simulink model "Vehicle_definitivo_validazione_2"  (R2025b)
settings: Solver=ode4  StartTime=0.0  StopTime=30  FixedStep=0.001  RelTol=1e-3
undefined symbols (not defined in the file): car, new_lotus_bump, new_lotus_roll, new_lotus_steer, posRef, rad, s, Tau_1, Tau_2, Tau_3, Tau_4, yawRef
libraries: aerolibconvert2 x28, simulink_extras x16, simulink x12, slpidlib x2, mpclib x1
(part 5 of 13)

== system Vehicle_definitivo_validazione_2/Torque Vectoring/Vehicle/Powertrain/Electric Motor ==
  T_target : Inport
  omega wheels : Inport  Port=2
  Angular Velocity Conversion : aerolibconvert2/Angular Velocity Conversion  IU=rpm  OU=rad/s
  Angular Velocity Conversion1 : aerolibconvert2/Angular Velocity Conversion  IU=rad/s  OU=rpm
  Angular Velocity Conversion2 : aerolibconvert2/Angular Velocity Conversion  IU=rpm  OU=rad/s
  Demux : Demux
  Gain1 : Gain  Gain=car.Tau_EM
  Gain2 : Gain  Gain=car.Tau_EM
  Gain3 : Gain  Gain=car.Tau_EM
  Integrator : Integrator  InitialCondition=1  LimitOutput=on  UpperSaturationLimit=1  LowerSaturationLimit=0
  Limiter1 : Saturate  UpperLimit=16000  LowerLimit=0
  MATLAB Function : MATLAB Function  TreatAsAtomicUnit=on
  MATLAB Function1 : MATLAB Function  TreatAsAtomicUnit=on
  Torque+ : Lookup_n-D  NumberOfTableDimensions=1  BreakpointsForDimension1=[0;5415.9399999999996;5455.8699999999999;5494.6300000000001;5524.8000000000002;5801.2200000000003;6194.8599999999997;6620.2799999999997;6996.5;7478.6599999999999;8072.5500000000002;8891.9799999999996;8998.9200000000001;9966.8600000000006;10994.200000000001;11872.6;13016.16;13972.65;15994.85]  Table=[6.914188;6.910217;6.868869;6.845731;6.823144;6.614154;6.313463;6.000783;5.723209;5.399066;4.994964;4.498184;4.450257;3.941032;3.52511;3.198601;2.816719;2.558901;2.040423]  InternalRulePriority=Speed  RndMeth=Simplest
  Torque+1 : Lookup_n-D  NumberOfTableDimensions=1  BreakpointsForDimension1=[0;5415.9399999999996;5455.8699999999999;5494.6300000000001;5524.8000000000002;5801.2200000000003;6194.8599999999997;6620.2799999999997;6996.5;7478.6599999999999;8072.5500000000002;8891.9799999999996;8998.9200000000001;9966.8600000000006;10994.200000000001;11872.6;13016.16;13972.65;15994.85]  Table=[6.914188;6.910217;6.868869;6.845731;6.823144;6.614154;6.313463;6.000783;5.723209;5.399066;4.994964;4.498184;4.450257;3.941032;3.52511;3.198601;2.816719;2.558901;2.040423]  InternalRulePriority=Speed  RndMeth=Simplest
  Torque- : Lookup_n-D  NumberOfTableDimensions=1  BreakpointsForDimension1=[0;5415.9399999999996;5455.8699999999999;5494.6300000000001;5524.8000000000002;5801.2200000000003;6194.8599999999997;6620.2799999999997;6996.5;7478.6599999999999;8072.5500000000002;8891.9799999999996;8998.9200000000001;9966.8600000000006;10994.200000000001;11872.6;13016.16;13972.65;15994.85]  Table=-[6.914188;6.910217;6.868869;6.845731;6.823144;6.614154;6.313463;6.000783;5.723209;5.399066;4.994964;4.498184;4.450257;3.941032;3.52511;3.198601;2.816719;2.558901;2.040423]  InternalRulePriority=Speed  RndMeth=Simplest
  Torque-1 : Lookup_n-D  NumberOfTableDimensions=1  BreakpointsForDimension1=[0;5415.9399999999996;5455.8699999999999;5494.6300000000001;5524.8000000000002;5801.2200000000003;6194.8599999999997;6620.2799999999997;6996.5;7478.6599999999999;8072.5500000000002;8891.9799999999996;8998.9200000000001;9966.8600000000006;10994.200000000001;11872.6;13016.16;13972.65;15994.85]  Table=-[6.914188;6.910217;6.868869;6.845731;6.823144;6.614154;6.313463;6.000783;5.723209;5.399066;4.994964;4.498184;4.450257;3.941032;3.52511;3.198601;2.816719;2.558901;2.040423]  InternalRulePriority=Speed  RndMeth=Simplest
  T_FR : Outport
  T_FL : Outport  Port=2
  wires:
  omega wheels/1 -> Angular Velocity Conversion1/1
  Angular Velocity Conversion1/1 -> Gain3/1
  Gain3/1 -> Limiter1/1
  Limiter1/1 -> Demux/1
  Demux/1 -> Torque+/1, Torque-/1, Angular Velocity Conversion/1
  Demux/2 -> Torque-1/1, Angular Velocity Conversion2/1, Torque+1/1
  MATLAB Function/1(SoC_dot) -> Integrator/1
  Integrator/1 -> MATLAB Function/5(SoC)
  Angular Velocity Conversion/1 -> MATLAB Function/3(w_FR)
  Angular Velocity Conversion2/1 -> MATLAB Function/4(w_FL)
  Torque+/1 -> MATLAB Function1/2(T_max_pos_FR)  "T_FR+"
  Torque+1/1 -> MATLAB Function1/4(T_max_pos_FL)  "T_FL+"
  Torque-/1 -> MATLAB Function1/3(T_max_neg_FR)  "T_FR-"
  Torque-1/1 -> MATLAB Function1/5(T_max_neg_FL)  "T_FL-"
  T_target/1 -> MATLAB Function1/1(T_target)
  MATLAB Function1/2(T_actual_FL) -> Gain2/1, MATLAB Function/2(T_FL)
  MATLAB Function1/1(T_actual_FR) -> Gain1/1, MATLAB Function/1(T_FR)
  Gain1/1 -> T_FR/1
  Gain2/1 -> T_FL/1

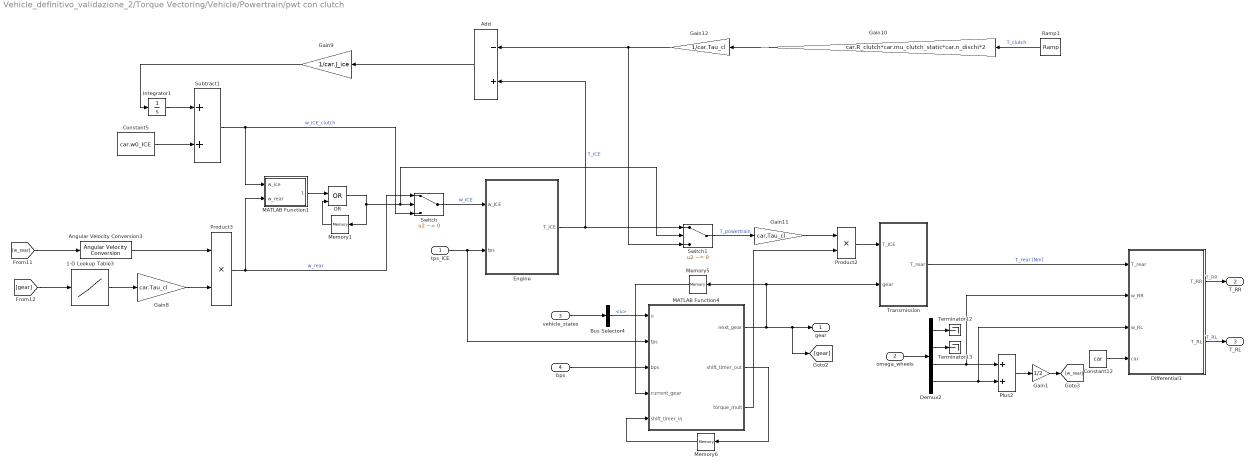
== system Vehicle_definitivo_validazione_2/Torque Vectoring/Vehicle/Powertrain/pwt con clutch ==
  tps_ICE : Inport
  omega_wheels : Inport  Port=2
  vehicle_states : Inport  Port=3
  bps : Inport  Port=4
  1-D Lookup Table3 : Lookup_n-D  NumberOfTableDimensions=1  BreakpointsForDimension1=[1;2;3;4]  Table=[Tau_1; Tau_2; Tau_3; Tau_4]  InternalRulePriority=Speed  RndMeth=Simplest
  Add : Sum  Inputs=-+
  Angular Velocity Conversion3 : aerolibconvert2/Angular Velocity Conversion  IU=rad/s  OU=rpm
  Bus Selector4 : BusSelector  OutputSignals=velocities.u
  Constant12 : Constant  Value=car  OutDataTypeStr=Bus: slBus1
  Constant5 : Constant  Value=car.w0_ICE
  Demux2 : Demux
  Differential1 : MATLAB Function  TreatAsAtomicUnit=on
  Engine : Subsystem
  Gain1 : Gain  Gain=1/2
  Gain10 : Gain  Gain=car.R_clutch*car.mu_clutch_static*car.n_dischi*2
  Gain11 : Gain  Gain=car.Tau_cl
  Gain12 : Gain  Gain=1/car.Tau_cl
  Gain8 : Gain  Gain=car.Tau_cl
  Gain9 : Gain  Gain=1/car.J_ice
  Integrator1 : Integrator
  MATLAB Function1 : MATLAB Function  TreatAsAtomicUnit=on
  MATLAB Function4 : MATLAB Function  TreatAsAtomicUnit=on
  Memory1 : Memory
  Memory5 : Memory  InitialCondition=2
  Memory6 : Memory
  OR : Logic  Operator=OR  IconShape=distinctive  AllPortsSameDT=off  OutDataTypeStr=boolean
  Plus2 : Sum
  Product2 : Product
  Product3 : Product
  Ramp1 : simulink/Sources/Ramp  slope=5000  start=0  InitialOutput=671
  Subtract1 : Sum
  Switch : Switch  Criteria=u2 ~= 0  Threshold=50  SaturateOnIntegerOverflow=off  InputSameDT=off
  Switch1 : Switch  Criteria=u2 ~= 0  Threshold=50  SaturateOnIntegerOverflow=off  InputSameDT=off
  Terminator12 : Terminator
  Terminator13 : Terminator
  Transmission : Subsystem
  gear : Outport
  T_RR : Outport  Port=2
  T_RL : Outport  Port=3
  wires:
  Ramp1/1 -> Gain10/1  "T_clutch"
  MATLAB Function1/1(condizione) -> OR/1
  [gear] -> 1-D Lookup Table3/1
  Gain10/1 -> Gain12/1
  Angular Velocity Conversion3/1 -> Product3/1
  [w_rear] -> Angular Velocity Conversion3/1
  Gain12/1 -> Switch1/3, Add/1
  Integrator1/1 -> Subtract1/1
  Switch/1 -> Engine/1(w_ICE)  "w_ICE"
  Subtract1/1 -> Switch/3, MATLAB Function1/1(w_ice)  "w_ICE_clutch"
  Switch1/1 -> Gain11/1  "T_powertrain"
  Constant5/1 -> Subtract1/2
  Memory1/1 -> OR/2
  tps_ICE/1 -> Engine/2(tps), MATLAB Function4/2(tps)
  Add/1 -> Gain9/1
  Memory5/1 -> MATLAB Function4/4(current_gear)
  bps/1 -> MATLAB Function4/3(bps)
  OR/1 -> Memory1/1, Switch/2, Switch1/2
  vehicle_states/1 -> Bus Selector4/1
  Demux2/1 -> Terminator12/1
  Gain8/1 -> Product3/2
  Gain1/1 -> [w_rear]
  1-D Lookup Table3/1 -> Gain8/1
  Plus2/1 -> Gain1/1
  omega_wheels/1 -> Demux2/1
  MATLAB Function4/2(shift_timer_out) -> Memory6/1
  Transmission/1(T_rear) -> Differential1/1(T_rear)  "T_rear [Nm]"
  Memory6/1 -> MATLAB Function4/5(shift_timer_in)
  Demux2/2 -> Terminator13/1
  Demux2/4 -> Differential1/3(w_RL), Plus2/2
  Bus Selector4/1 -> MATLAB Function4/1(u)  "<u>"
  Demux2/3 -> Differential1/2(w_RR), Plus2/1
  MATLAB Function4/1(next_gear) -> Memory5/1, Transmission/2(gear), gear/1, [gear]
  Product3/1 -> MATLAB Function1/2(w_rear), Switch/1  "w_rear"
  Gain11/1 -> Product2/1
  MATLAB Function4/3(torque_mult) -> Product2/2
  Engine/1(T_ICE) -> Add/2, Switch1/1  "T_ICE"
  Gain9/1 -> Integrator1/1
  Product2/1 -> Transmission/1(T_ICE)
  Differential1/1(T_RR) -> T_RR/1  "T_RR"
  Constant12/1 -> Differential1/4(car)
  Differential1/2(T_RL) -> T_RL/1  "T_RL"

== system Vehicle_definitivo_validazione_2/Torque Vectoring/Vehicle/Powertrain/pwt senza clutch ==
  tps_ICE : Inport
  vehicle_states : Inport  Port=2
  bps : Inport  Port=3
  omega_wheels : Inport  Port=4
  1-D Lookup Table1 : Lookup_n-D  NumberOfTableDimensions=1  BreakpointsForDimension1=[1;2;3;4]  Table=[Tau_1; Tau_2; Tau_3; Tau_4]  InternalRulePriority=Speed  RndMeth=Simplest
  Angular Velocity Conversion1 : aerolibconvert2/Angular Velocity Conversion  IU=rad/s  OU=rpm
  Bus Selector3 : BusSelector  OutputSignals=Veh_States.velocities.u
  Constant12 : Constant  Value=car  OutDataTypeStr=Bus: slBus1
  Demux : Demux
  Differential : MATLAB Function  TreatAsAtomicUnit=on
  Engine : Subsystem
  Gain1 : Gain  Gain=1/2
  Gain2 : Gain  Gain=car.Tau_cl
  Gain5 : Gain  Gain=car.Tau_cl
  Gearbox : MATLAB Function  TreatAsAtomicUnit=on
  Memory : Memory  InitialCondition=2
  Memory3 : Memory
  Plus : Sum
  Product : Product
  Product1 : Product
  Terminator : Terminator
  Terminator1 : Terminator
  Transmission : Subsystem
  T_RR : Outport
  T_RL : Outport  Port=2
  gear : Outport  Port=3
  wires:
  Memory/1 -> Gearbox/4(current_gear)
  Gain5/1 -> Product1/2
  vehicle_states/1 -> Bus Selector3/1
  Angular Velocity Conversion1/1 -> Product1/1
  Gearbox/3(shift_timer_out) -> Memory3/1
  Memory3/1 -> Gearbox/5(shift_timer_in)
  bps/1 -> Gearbox/3(bps)  "bps"
  1-D Lookup Table1/1 -> Gain5/1
  Bus Selector3/1 -> Gearbox/1(u)  "<u>"
  Gearbox/1(next_gear) -> Memory/1, Transmission/2(gear), gear/1, [gear]  "gear"
  [gear] -> 1-D Lookup Table1/1
  Transmission/1(T_rear) -> Differential/1(T_rear)  "T_rear [Nm]"
  tps_ICE/1 -> Gearbox/2(tps), Engine/2(tps)  "tps"
  Product/1 -> Transmission/1(T_ICE)
  Engine/1(T_ICE) -> Gain2/1  "T_ICE"
  Product1/1 -> Engine/1(w_ICE)  "w_ICE"
  Gearbox/2(torque_mult) -> Product/2
  Gain2/1 -> Product/1
  Plus/1 -> Gain1/1
  Demux/3 -> Plus/1, [w_RR]
  Gain1/1 -> Angular Velocity Conversion1/1
  Demux/4 -> [w_RL], Plus/2
  omega_wheels/1 -> Demux/1
  Demux/1 -> Terminator/1  "w_front"
  Demux/2 -> Terminator1/1
  Differential/1(T_RR) -> T_RR/1  "T_RR"
  Differential/2(T_RL) -> T_RL/1  "T_RL"
  [w_RR] -> Differential/2(w_RR)
  [w_RL] -> Differential/3(w_RL)
  Constant12/1 -> Differential/4(car)

== system Vehicle_definitivo_validazione_2/Torque Vectoring/Vehicle/Powertrain con differenziale1/Electric Motor ==
  tps_EM : Inport
  omega wheels : Inport  Port=2
  2-D Lookup Table : Lookup_n-D  BreakpointsForDimension1=[0;5415.9399999999996;5455.8699999999999;5494.6300000000001;5524.8000000000002;5801.2200000000003;6194.8599999999997;6620.2799999999997;6996.5;7478.6599999999999;8072.5500000000002;8891.9799999999996;8998.9200000000001;9966.8600000000006;10994.200000000001;11872.6;13016.16;13972.65;15994.85]  BreakpointsForDimension2=[0;0.25;0.29999999999999999;0.34999999999999998;0.40000000000000002;0.45000000000000001;0.5;0.59999999999999998;0.69999999999999996;0.80000000000000004;1]  Table=[0 1.72854705 2.07425646 2.41996587 2.7656752899999999 3.1113846999999999 3.4570941099999999 4.1485129299999999 4.8399317000000002 5.5313505699999999 6.9141880000000002;0 1.72755429 2.0730651500000001 2.4185760100000002 2.7640868599999999 3.10959772 3.4551085800000001 4.1461303000000003 4.8371519999999997 5.5281737299999998 6.9102170000000003;0 1.7172173399999999 2.0606608099999999 2.4041042799999999 2.7475477499999998 3.0909912099999999 3.4344346799999999 4.1213216199999998 4.8082086000000004 5.4950954899999997 6.8688690000000001;0 1.7114327 2.0537192399999999 2.3960057799999999 2.7382923199999998 3.0805788600000001 3.4228654000000001 4.1074384799999999 4.7920116000000004 5.4765846399999996 6.8457309999999998;0 1.7057860899999999 2.0469433100000001 2.3881005200000001 2.72925774 3.0704149599999999 3.4115721799999998 4.0938866100000002 4.7762010000000004 5.45851548 6.8231440000000001;0 1.65353861 1.9842463299999999 2.3149540499999999 2.6456617699999998 2.9763694900000002 3.3070772100000001 3.96849265 4.6299080999999997 5.2913235399999996 6.6141540000000001;0 1.57836584 1.89403901 2.2097121799999999 2.5253853500000001 2.8410585199999998 3.15673168 3.7880780199999999 4.4194243999999996 5.0507707000000002 6.3134629999999996;0 1.5001957400000001 1.80023489 2.10027404 2.4003131899999999 2.7003523399999998 3.0003914800000002 3.6004697800000001 4.2005480999999998 4.8006263699999998 6.0007830000000002;0 1.43080228 1.71696274 2.0031231900000002 2.2892836499999998 2.5754440999999999 2.86160456 3.4339254700000001 4.0062464000000002 4.5785672899999996 5.7232089999999998;0 1.34976662 1.6197199499999999 1.8896732700000001 2.1596266000000002 2.4295799200000001 2.69953325 3.2394398899999999 3.7793464999999999 4.3192531900000004 5.3990660000000004;0 1.24874098 1.49848917 1.74823737 1.99798556 2.24773376 2.4974819500000001 2.9969783400000001 3.4964746999999998 3.9959711200000001 4.9949640000000004;0 1.1245459799999999 1.3494551800000001 1.57436438 1.79927357 2.0241827699999999 2.2490919699999998 2.6989103600000002 3.1487288000000002 3.5985471499999999 4.4981840000000002;0 1.11256427 1.3350771299999999 1.5575899799999999 1.7801028299999999 2.0026156899999998 2.22512854 2.67015425 3.1151800000000001 3.5602056700000002 4.4502569999999997;0 0.98525799000000003 1.18230959 1.3793611800000001 1.5764127800000001 1.7734643800000001 1.9705159800000001 2.3646191700000001 2.7587223999999999 3.1528255600000001 3.9410319999999999;0 0.88127745999999996 1.0575329600000001 1.23378845 1.41004394 1.5862994399999999 1.7625549300000001 2.1150659100000002 2.4675769000000001 2.8200878899999999 3.5251100000000002;0 0.79965012999999996 0.95958014999999997 1.11951018 1.2794402 1.43937023 1.59930025 1.9191602999999999 2.2390203999999998 2.5588804000000001 3.198601;0 0.70417978000000003 0.84501572999999996 0.98585168999999995 1.1266876400000001 1.2675236000000001 1.4083595600000001 1.6900314700000001 1.9717034 2.2533752900000001 2.816719;0 0.63972525999999996 0.76767032000000002 0.89561537000000002 1.0235604199999999 1.15150547 1.2794505300000001 1.5353406300000001 1.7912307000000001 2.0471208399999998 2.5589010000000001;0 0.51010575999999996 0.61212690999999997 0.71414805999999997 0.81616922000000003 0.91819037000000003 1.0202115199999999 1.2242538199999999 1.4282961000000001 1.6323384299999999 2.0404230000000001]  InternalRulePriority=Speed  RndMeth=Simplest
      settings: InputPortMap=u0,u1
  2-D Lookup Table1 : Lookup_n-D  BreakpointsForDimension1=[0;5415.9399999999996;5455.8699999999999;5494.6300000000001;5524.8000000000002;5801.2200000000003;6194.8599999999997;6620.2799999999997;6996.5;7478.6599999999999;8072.5500000000002;8891.9799999999996;8998.9200000000001;9966.8600000000006;10994.200000000001;11872.6;13016.16;13972.65;15994.85]  BreakpointsForDimension2=[0;0.25;0.29999999999999999;0.34999999999999998;0.40000000000000002;0.45000000000000001;0.5;0.59999999999999998;0.69999999999999996;0.80000000000000004;1]  Table=[0 1.72854705 2.07425646 2.41996587 2.7656752899999999 3.1113846999999999 3.4570941099999999 4.1485129299999999 4.8399317000000002 5.5313505699999999 6.9141880000000002;0 1.72755429 2.0730651500000001 2.4185760100000002 2.7640868599999999 3.10959772 3.4551085800000001 4.1461303000000003 4.8371519999999997 5.5281737299999998 6.9102170000000003;0 1.7172173399999999 2.0606608099999999 2.4041042799999999 2.7475477499999998 3.0909912099999999 3.4344346799999999 4.1213216199999998 4.8082086000000004 5.4950954899999997 6.8688690000000001;0 1.7114327 2.0537192399999999 2.3960057799999999 2.7382923199999998 3.0805788600000001 3.4228654000000001 4.1074384799999999 4.7920116000000004 5.4765846399999996 6.8457309999999998;0 1.7057860899999999 2.0469433100000001 2.3881005200000001 2.72925774 3.0704149599999999 3.4115721799999998 4.0938866100000002 4.7762010000000004 5.45851548 6.8231440000000001;0 1.65353861 1.9842463299999999 2.3149540499999999 2.6456617699999998 2.9763694900000002 3.3070772100000001 3.96849265 4.6299080999999997 5.2913235399999996 6.6141540000000001;0 1.57836584 1.89403901 2.2097121799999999 2.5253853500000001 2.8410585199999998 3.15673168 3.7880780199999999 4.4194243999999996 5.0507707000000002 6.3134629999999996;0 1.5001957400000001 1.80023489 2.10027404 2.4003131899999999 2.7003523399999998 3.0003914800000002 3.6004697800000001 4.2005480999999998 4.8006263699999998 6.0007830000000002;0 1.43080228 1.71696274 2.0031231900000002 2.2892836499999998 2.5754440999999999 2.86160456 3.4339254700000001 4.0062464000000002 4.5785672899999996 5.7232089999999998;0 1.34976662 1.6197199499999999 1.8896732700000001 2.1596266000000002 2.4295799200000001 2.69953325 3.2394398899999999 3.7793464999999999 4.3192531900000004 5.3990660000000004;0 1.24874098 1.49848917 1.74823737 1.99798556 2.24773376 2.4974819500000001 2.9969783400000001 3.4964746999999998 3.9959711200000001 4.9949640000000004;0 1.1245459799999999 1.3494551800000001 1.57436438 1.79927357 2.0241827699999999 2.2490919699999998 2.6989103600000002 3.1487288000000002 3.5985471499999999 4.4981840000000002;0 1.11256427 1.3350771299999999 1.5575899799999999 1.7801028299999999 2.0026156899999998 2.22512854 2.67015425 3.1151800000000001 3.5602056700000002 4.4502569999999997;0 0.98525799000000003 1.18230959 1.3793611800000001 1.5764127800000001 1.7734643800000001 1.9705159800000001 2.3646191700000001 2.7587223999999999 3.1528255600000001 3.9410319999999999;0 0.88127745999999996 1.0575329600000001 1.23378845 1.41004394 1.5862994399999999 1.7625549300000001 2.1150659100000002 2.4675769000000001 2.8200878899999999 3.5251100000000002;0 0.79965012999999996 0.95958014999999997 1.11951018 1.2794402 1.43937023 1.59930025 1.9191602999999999 2.2390203999999998 2.5588804000000001 3.198601;0 0.70417978000000003 0.84501572999999996 0.98585168999999995 1.1266876400000001 1.2675236000000001 1.4083595600000001 1.6900314700000001 1.9717034 2.2533752900000001 2.816719;0 0.63972525999999996 0.76767032000000002 0.89561537000000002 1.0235604199999999 1.15150547 1.2794505300000001 1.5353406300000001 1.7912307000000001 2.0471208399999998 2.5589010000000001;0 0.51010575999999996 0.61212690999999997 0.71414805999999997 0.81616922000000003 0.91819037000000003 1.0202115199999999 1.2242538199999999 1.4282961000000001 1.6323384299999999 2.0404230000000001]  InternalRulePriority=Speed  RndMeth=Simplest
      settings: InputPortMap=u0,u1
  Angular Velocity Conversion1 : aerolibconvert2/Angular Velocity Conversion  IU=rad/s  OU=rpm
  Demux : Demux
  Gain : Gain  Gain=car.Tau_EM
  Gain1 : Gain  Gain=car.Tau_EM
  Gain3 : Gain  Gain=car.Tau_EM
  Limiter1 : Saturate  UpperLimit=16000  LowerLimit=0
  T_FR : Outport
  T_FL : Outport  Port=2
  wires:
  Demux/2 -> 2-D Lookup Table1/1
  Demux/1 -> 2-D Lookup Table/1
  Limiter1/1 -> Demux/1
  tps_EM/1 -> 2-D Lookup Table/2, 2-D Lookup Table1/2
  Gain1/1 -> T_FL/1
  Gain/1 -> T_FR/1
  Gain3/1 -> Limiter1/1
  Angular Velocity Conversion1/1 -> Gain3/1
  omega wheels/1 -> Angular Velocity Conversion1/1
  2-D Lookup Table1/1 -> Gain1/1
  2-D Lookup Table/1 -> Gain/1

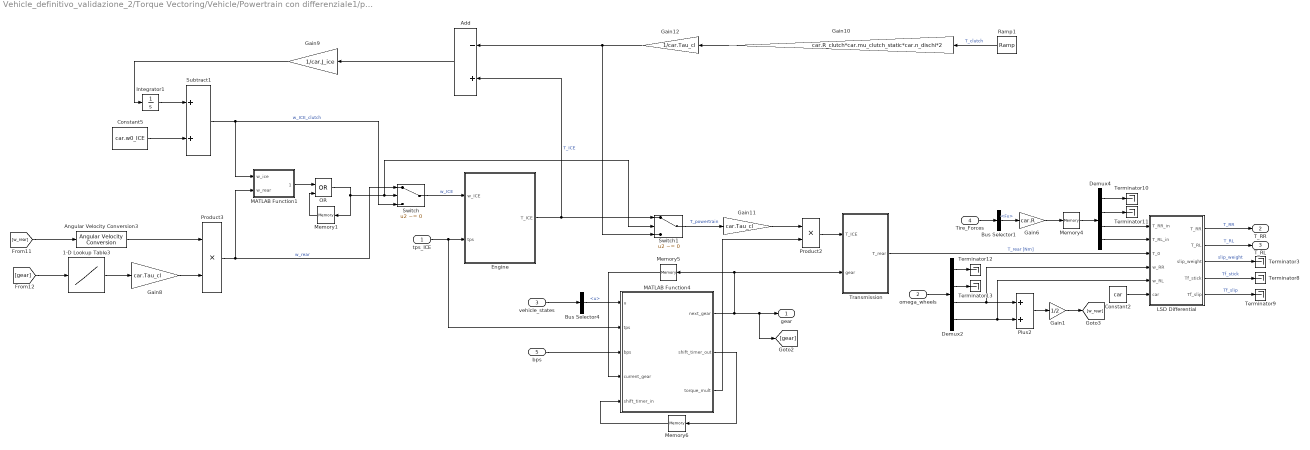
== system Vehicle_definitivo_validazione_2/Torque Vectoring/Vehicle/Powertrain con differenziale1/pwt con clutch ==
  tps_ICE : Inport
  omega_wheels : Inport  Port=2
  vehicle_states : Inport  Port=3
  Tire_Forces : Inport  Port=4
  bps : Inport  Port=5
  1-D Lookup Table3 : Lookup_n-D  NumberOfTableDimensions=1  BreakpointsForDimension1=[1;2;3;4]  Table=[Tau_1; Tau_2; Tau_3; Tau_4]  InternalRulePriority=Speed  RndMeth=Simplest
  Add : Sum  Inputs=-+
  Angular Velocity Conversion3 : aerolibconvert2/Angular Velocity Conversion  IU=rad/s  OU=rpm
  Bus Selector1 : BusSelector  OutputSignals=Fx
  Bus Selector4 : BusSelector  OutputSignals=velocities.u
  Constant2 : Constant  Value=car  OutDataTypeStr=Bus: slBus1
  Constant5 : Constant  Value=car.w0_ICE
  Demux2 : Demux
  Demux4 : Demux
  Engine : Subsystem
  Gain1 : Gain  Gain=1/2
  Gain10 : Gain  Gain=car.R_clutch*car.mu_clutch_static*car.n_dischi*2
  Gain11 : Gain  Gain=car.Tau_cl
  Gain12 : Gain  Gain=1/car.Tau_cl
  Gain6 : Gain  Gain=car.R
  Gain8 : Gain  Gain=car.Tau_cl
  Gain9 : Gain  Gain=1/car.J_ice
  Integrator1 : Integrator
  LSD Differential : MATLAB Function  TreatAsAtomicUnit=on
  MATLAB Function1 : MATLAB Function  TreatAsAtomicUnit=on
  MATLAB Function4 : MATLAB Function  TreatAsAtomicUnit=on
  Memory1 : Memory
  Memory4 : Memory
  Memory5 : Memory  InitialCondition=2
  Memory6 : Memory
  OR : Logic  Operator=OR  IconShape=distinctive  AllPortsSameDT=off  OutDataTypeStr=boolean
  Plus2 : Sum
  Product2 : Product
  Product3 : Product
  Ramp1 : simulink/Sources/Ramp  slope=5000  start=0  InitialOutput=671
  Subtract1 : Sum
  Switch : Switch  Criteria=u2 ~= 0  Threshold=50  SaturateOnIntegerOverflow=off  InputSameDT=off
  Switch1 : Switch  Criteria=u2 ~= 0  Threshold=50  SaturateOnIntegerOverflow=off  InputSameDT=off
  Terminator{3,8..13} (7 alike) : Terminator
  Transmission : Subsystem
  gear : Outport
  T_RR : Outport  Port=2
  T_RL : Outport  Port=3
  wires:
  Product2/1 -> Transmission/1(T_ICE)
  Demux4/1 -> Terminator10/1
  Gain9/1 -> Integrator1/1
  Engine/1(T_ICE) -> Switch1/1, Add/2  "T_ICE"
  MATLAB Function4/3(torque_mult) -> Product2/2
  Gain11/1 -> Product2/1
  LSD Differential/1(T_RR) -> T_RR/1  "T_RR"
  Product3/1 -> Switch/1, MATLAB Function1/2(w_rear)  "w_rear"
  Tire_Forces/1 -> Bus Selector1/1
  LSD Differential/4(Tf_stick) -> Terminator8/1  "Tf_stick"
  MATLAB Function4/1(next_gear) -> [gear], gear/1, Transmission/2(gear), Memory5/1
  Demux2/3 -> LSD Differential/4(w_RR), Plus2/1
  Bus Selector4/1 -> MATLAB Function4/1(u)  "<u>"
  Gain6/1 -> Memory4/1
  LSD Differential/5(Tf_slip) -> Terminator9/1  "Tf_slip"
  Demux4/4 -> LSD Differential/2(T_RL_in)
  LSD Differential/3(slip_weight) -> Terminator3/1  "slip_weight"
  Demux2/4 -> LSD Differential/5(w_RL), Plus2/2
  LSD Differential/2(T_RL) -> T_RL/1  "T_RL"
  Demux2/2 -> Terminator13/1
  Memory4/1 -> Demux4/1
  Constant2/1 -> LSD Differential/6(car)
  Memory6/1 -> MATLAB Function4/5(shift_timer_in)
  Demux4/3 -> LSD Differential/1(T_RR_in)
  Transmission/1(T_rear) -> LSD Differential/3(T_0)  "T_rear [Nm]"
  Bus Selector1/1 -> Gain6/1  "<Fx>"
  Demux4/2 -> Terminator11/1
  MATLAB Function4/2(shift_timer_out) -> Memory6/1
  omega_wheels/1 -> Demux2/1
  Plus2/1 -> Gain1/1
  1-D Lookup Table3/1 -> Gain8/1
  Gain1/1 -> [w_rear]
  Gain8/1 -> Product3/2
  Demux2/1 -> Terminator12/1
  vehicle_states/1 -> Bus Selector4/1
  OR/1 -> Switch1/2, Switch/2, Memory1/1
  bps/1 -> MATLAB Function4/3(bps)
  Memory5/1 -> MATLAB Function4/4(current_gear)
  Add/1 -> Gain9/1
  tps_ICE/1 -> MATLAB Function4/2(tps), Engine/2(tps)
  Memory1/1 -> OR/2
  Constant5/1 -> Subtract1/2
  Switch1/1 -> Gain11/1  "T_powertrain"
  Subtract1/1 -> MATLAB Function1/1(w_ice), Switch/3  "w_ICE_clutch"
  Switch/1 -> Engine/1(w_ICE)  "w_ICE"
  Integrator1/1 -> Subtract1/1
  Gain12/1 -> Add/1, Switch1/3
  [w_rear] -> Angular Velocity Conversion3/1
  Angular Velocity Conversion3/1 -> Product3/1
  Gain10/1 -> Gain12/1
  [gear] -> 1-D Lookup Table3/1
  MATLAB Function1/1(condizione) -> OR/1
  Ramp1/1 -> Gain10/1  "T_clutch"

== system Vehicle_definitivo_validazione_2/Torque Vectoring/Vehicle/Powertrain con differenziale1/pwt senza clutch ==
  tps_ICE : Inport
  omega_wheels : Inport  Port=2
  vehicle_states : Inport  Port=3
  Tire_Forces : Inport  Port=4
  bps : Inport  Port=5
  1-D Lookup Table1 : Lookup_n-D  NumberOfTableDimensions=1  BreakpointsForDimension1=[1;2;3;4]  Table=[Tau_1; Tau_2; Tau_3; Tau_4]  InternalRulePriority=Speed  RndMeth=Simplest
  Angular Velocity Conversion1 : aerolibconvert2/Angular Velocity Conversion  IU=rad/s  OU=rpm
  Bus Selector2 : BusSelector  OutputSignals=Fx
  Bus Selector3 : BusSelector  OutputSignals=velocities.u
  Constant1 : Constant  Value=car  OutDataTypeStr=Bus: slBus1
  Demux1 : Demux
  Demux3 : Demux
  Engine : Subsystem
  Gain2 : Gain  Gain=1/2
  Gain3 : Gain  Gain=car.R
  Gain4 : Gain  Gain=car.Tau_cl
  Gain5 : Gain  Gain=car.Tau_cl
  LSD Differential : MATLAB Function  TreatAsAtomicUnit=on
  MATLAB Function3 : MATLAB Function  TreatAsAtomicUnit=on
  Memory : Memory  InitialCondition=2
  Memory2 : Memory
  Memory3 : Memory
  Plus1 : Sum
  Product : Product
  Product1 : Product
  Terminator{,1..2,4..7} (7 alike) : Terminator
  Transmission : Subsystem
  T_RR : Outport
  T_RL : Outport  Port=2
  gear : Outport  Port=3
  wires:
  Gain4/1 -> Product/1
  MATLAB Function3/3(torque_mult) -> Product/2
  Product1/1 -> Engine/1(w_ICE)  "w_ICE"
  LSD Differential/4(Tf_stick) -> Terminator1/1  "Tf_stick"
  LSD Differential/5(Tf_slip) -> Terminator2/1  "Tf_slip"
  LSD Differential/3(slip_weight) -> Terminator/1  "slip_weight"
  Demux1/3 -> LSD Differential/4(w_RR), Plus1/1
  Engine/1(T_ICE) -> Gain4/1  "T_ICE"
  Demux1/4 -> LSD Differential/5(w_RL), Plus1/2
  Demux3/4 -> LSD Differential/2(T_RL_in)
  Demux1/2 -> Terminator7/1
  omega_wheels/1 -> Demux1/1
  Product/1 -> Transmission/1(T_ICE)
  [w_rear] -> Angular Velocity Conversion1/1
  Tire_Forces/1 -> Bus Selector2/1
  LSD Differential/2(T_RL) -> T_RL/1  "T_RL"
  Demux3/3 -> LSD Differential/1(T_RR_in)
  tps_ICE/1 -> Engine/2(tps), MATLAB Function3/2(tps)  "tps"
  Transmission/1(T_rear) -> LSD Differential/3(T_0)  "T_rear [Nm]"
  LSD Differential/1(T_RR) -> T_RR/1  "T_RR"
  [gear] -> 1-D Lookup Table1/1
  MATLAB Function3/1(next_gear) -> [gear], gear/1, Transmission/2(gear), Memory/1  "gear"
  Gain2/1 -> [w_rear]
  Bus Selector3/1 -> MATLAB Function3/1(u)  "<u>"
  Memory2/1 -> Demux3/1
  Constant1/1 -> LSD Differential/6(car)
  Demux3/1 -> Terminator4/1
  1-D Lookup Table1/1 -> Gain5/1
  Gain3/1 -> Memory2/1
  bps/1 -> MATLAB Function3/3(bps)  "bps"
  Memory3/1 -> MATLAB Function3/5(shift_timer_in)
  MATLAB Function3/2(shift_timer_out) -> Memory3/1
  Bus Selector2/1 -> Gain3/1  "<Fx>"
  Angular Velocity Conversion1/1 -> Product1/1
  Plus1/1 -> Gain2/1
  vehicle_states/1 -> Bus Selector3/1
  Gain5/1 -> Product1/2
  Demux3/2 -> Terminator5/1
  Memory/1 -> MATLAB Function3/4(current_gear)
  Demux1/1 -> Terminator6/1

== system Vehicle_definitivo_validazione_2/Con relaxation/Vehicle/Chassis/Damper/FL ==
  V_FL : Inport
  Add : Sum
  Add1 : Sum
  Add2 : Sum
  Front compression min : Lookup_n-D  NumberOfTableDimensions=1  BreakpointsForDimension1=|  Table=|  InternalRulePriority=Speed  RndMeth=Simplest
      BreakpointsForDimension1=|
      | [0;0.025;0.051;0.076;0.102;0.127;0.152;0.178;0.203;0.229;0.254;0.279;0.305
      | ]
      Table=|
      | [0; 240.204;
      | 231.307;
      | 226.859;
      | 226.859;
      | 231.307;
      | 231.307;
      | 235.756;
      | 240.204;
      | 240.204;
      | 244.652;
      | 249.100;
      | 253.549]
  Gain : Gain  Gain=-1
  Gain1 : Gain  Gain=-1
  Gain2 : Gain  Gain=car.click_comp_F/car.click_tot_comp_F
  Gain3 : Gain  Gain=car.click_reb_F/car.click_tot_reb_F
  Saturation : Saturate  UpperLimit=inf  LowerLimit=0
  Saturation1 : Saturate  UpperLimit=0  LowerLimit=-inf
  Subtract : Sum  Inputs=+-
  Subtract1 : Sum  Inputs=+-
  front compression max : Lookup_n-D  NumberOfTableDimensions=1  BreakpointsForDimension1=|  Table=|  InternalRulePriority=Speed  RndMeth=Simplest
      BreakpointsForDimension1=|
      | [0;0.025;0.051;0.076;0.102;0.127;0.152;0.178;0.203;0.229;0.254;0.279;0.305
      | ]
      Table=|
      | [0;782.887;
      | 898.540;
      | 956.367;
      | 978.608;
      | 1000.850;
      | 1018.642;
      | 1058.676;
      | 1085.366;
      | 1107.607;
      | 1147.641
      | ;1178.778;1214.364
      | ]
  front rebound max : Lookup_n-D  NumberOfTableDimensions=1  BreakpointsForDimension1=|  Table=|  InternalRulePriority=Speed  RndMeth=Simplest
      BreakpointsForDimension1=|
      | [0;0.025;0.051;0.076;0.102;0.127;0.152;0.178;0.203;0.229;0.254;0.279;0.305
      | ]
      Table=|
      | [0; 266.893;
      | 333.617;
      | 360.306;
      | 373.650;
      | 391.443;
      | 409.236;
      | 422.581;
      | 444.822;
      | 467.063;
      | 480.408;
      | 493.752;
      | 511.545]
  front rebound min : Lookup_n-D  NumberOfTableDimensions=1  BreakpointsForDimension1=|  Table=|  InternalRulePriority=Speed  RndMeth=Simplest
      BreakpointsForDimension1=|
      | [0;0.025;0.051;0.076;0.102;0.127;0.152;0.178;0.203;0.229;0.254;0.279;0.305
      | ]
      Table=|
      | [0; 40.034;
      | 26.689;
      | 17.793;
      | 8.896;
      | 4.448;
      | 4.448;
      | 4.448;
      | 8.896;
      | 35.586;
      | 31.138;
      | 53.379;
      | 26.689]
  F_FL : Outport
  wires:
  Front compression min/1 -> Subtract/2, Add1/2
  front rebound min/1 -> Add2/2, Subtract1/2
  Subtract1/1 -> Gain3/1
  Gain3/1 -> Add2/1
  Subtract/1 -> Gain2/1
  Gain2/1 -> Add1/1
  front compression max/1 -> Subtract/1
  front rebound max/1 -> Subtract1/1
  Saturation/1 -> front compression max/1, Front compression min/1
  Gain1/1 -> front rebound min/1, front rebound max/1
  Add2/1 -> Gain/1
  V_FL/1 -> Saturation/1, Saturation1/1
  Saturation1/1 -> Gain1/1
  Gain/1 -> Add/2
  Add1/1 -> Add/1
  Add/1 -> F_FL/1

== system Vehicle_definitivo_validazione_2/Con relaxation/Vehicle/Chassis/Damper/FR ==
  V_FR : Inport
  Add : Sum
  Add1 : Sum
  Add2 : Sum
  Front compression min : Lookup_n-D  NumberOfTableDimensions=1  BreakpointsForDimension1=|  Table=|  InternalRulePriority=Speed  RndMeth=Simplest
      BreakpointsForDimension1=|
      | [0;0.025;0.051;0.076;0.102;0.127;0.152;0.178;0.203;0.229;0.254;0.279;0.305
      | ]
      Table=|
      | [0; 240.204;
      | 231.307;
      | 226.859;
      | 226.859;
      | 231.307;
      | 231.307;
      | 235.756;
      | 240.204;
      | 240.204;
      | 244.652;
      | 249.100;
      | 253.549]
  Gain : Gain  Gain=-1
  Gain1 : Gain  Gain=-1
  Gain2 : Gain  Gain=car.click_comp_F/car.click_tot_comp_F
  Gain3 : Gain  Gain=car.click_reb_F/car.click_tot_reb_F
  Saturation : Saturate  UpperLimit=inf  LowerLimit=0
  Saturation1 : Saturate  UpperLimit=0  LowerLimit=-inf
  Subtract : Sum  Inputs=+-
  Subtract1 : Sum  Inputs=+-
  front compression max : Lookup_n-D  NumberOfTableDimensions=1  BreakpointsForDimension1=|  Table=|  InternalRulePriority=Speed  RndMeth=Simplest
      BreakpointsForDimension1=|
      | [0;0.025;0.051;0.076;0.102;0.127;0.152;0.178;0.203;0.229;0.254;0.279;0.305
      | ]
      Table=|
      | [0;782.887;
      | 898.540;
      | 956.367;
      | 978.608;
      | 1000.850;
      | 1018.642;
      | 1058.676;
      | 1085.366;
      | 1107.607;
      | 1147.641
      | ;1178.778;1214.364
      | ]
  front rebound max : Lookup_n-D  NumberOfTableDimensions=1  BreakpointsForDimension1=|  Table=|  InternalRulePriority=Speed  RndMeth=Simplest
      BreakpointsForDimension1=|
      | [0;0.025;0.051;0.076;0.102;0.127;0.152;0.178;0.203;0.229;0.254;0.279;0.305
      | ]
      Table=|
      | [0; 266.893;
      | 333.617;
      | 360.306;
      | 373.650;
      | 391.443;
      | 409.236;
      | 422.581;
      | 444.822;
      | 467.063;
      | 480.408;
      | 493.752;
      | 511.545]
  front rebound min : Lookup_n-D  NumberOfTableDimensions=1  BreakpointsForDimension1=|  Table=|  InternalRulePriority=Speed  RndMeth=Simplest
      BreakpointsForDimension1=|
      | [0;0.025;0.051;0.076;0.102;0.127;0.152;0.178;0.203;0.229;0.254;0.279;0.305
      | ]
      Table=|
      | [0; 40.034;
      | 26.689;
      | 17.793;
      | 8.896;
      | 4.448;
      | 4.448;
      | 4.448;
      | 8.896;
      | 35.586;
      | 31.138;
      | 53.379;
      | 26.689]
  F_FR : Outport
  wires:
  Front compression min/1 -> Subtract/2, Add1/2
  front rebound min/1 -> Add2/2, Subtract1/2
  Subtract1/1 -> Gain3/1
  Gain3/1 -> Add2/1
  Subtract/1 -> Gain2/1
  Gain2/1 -> Add1/1
  front compression max/1 -> Subtract/1
  front rebound max/1 -> Subtract1/1
  Saturation/1 -> front compression max/1, Front compression min/1
  Gain1/1 -> front rebound min/1, front rebound max/1
  Add2/1 -> Gain/1
  V_FR/1 -> Saturation/1, Saturation1/1
  Saturation1/1 -> Gain1/1
  Gain/1 -> Add/2
  Add1/1 -> Add/1
  Add/1 -> F_FR/1

== system Vehicle_definitivo_validazione_2/Con relaxation/Vehicle/Chassis/Damper/RL ==
  V_RL : Inport
  Add : Sum
  Add1 : Sum
  Add2 : Sum
  Gain : Gain  Gain=-1
  Gain1 : Gain  Gain=-1
  Gain2 : Gain  Gain=car.click_comp_R/car.click_tot_comp_R
  Gain3 : Gain  Gain=car.click_reb_R/car.click_tot_reb_R
  Rear Compression max : Lookup_n-D  NumberOfTableDimensions=1  BreakpointsForDimension1=|  Table=|  InternalRulePriority=Speed  RndMeth=Simplest
      BreakpointsForDimension1=|
      | [0; 0.025;
      | 0.051;
      | 0.076;
      | 0.102;
      | 0.127;
      | 0.152;
      | 0.178;
      | 0.203;
      | 0.229;
      | 0.254;
      | 0.279;
      | 0.305
      | ]
      Table=|
      | [0; 667.233;
      | 782.887;
      | 885.196;
      | 934.126;
      | 965.264;
      | 996.401;
      | 1018.642;
      | 1049.780;
      | 1076.469;
      | 1112.055;
      | 1138.744;  1169.882
      | ]
  Rear Compression min : Lookup_n-D  NumberOfTableDimensions=1  BreakpointsForDimension1=|  Table=|  InternalRulePriority=Speed  RndMeth=Simplest
      BreakpointsForDimension1=|
      | [0; 0.025;
      | 0.051;
      | 0.076;
      | 0.102;
      | 0.127;
      | 0.152;
      | 0.178;
      | 0.203;
      | 0.229;
      | 0.254;
      | 0.279;
      | 0.305
      | ]
      Table=|
      | [0; 213.515;
      | 204.618;
      | 200.170;
      | 195.722;
      | 195.722;
      | 200.170;
      | 200.170;
      | 204.618;
      | 204.618;
      | 209.066;
      | 213.515;
      | 213.515
      | ]
  Rear Rebound max : Lookup_n-D  NumberOfTableDimensions=1  BreakpointsForDimension1=|  Table=|  InternalRulePriority=Speed  RndMeth=Simplest
      BreakpointsForDimension1=|
      | [0; 0.025;
      | 0.051;
      | 0.076;
      | 0.102;
      | 0.127;
      | 0.152;
      | 0.178;
      | 0.203;
      | 0.229;
      | 0.254;
      | 0.279;
      | 0.305
      | ]
      Table=|
      | [0; 124.550;
      | 191.273;
      | 244.652;
      | 284.686;
      | 329.168;
      | 369.202;
      | 391.443;
      | 413.684;
      | 431.477;
      | 449.270;
      | 458.167;
      | 471.511
      | ]
  Rear Rebound min : Lookup_n-D  NumberOfTableDimensions=1  BreakpointsForDimension1=|  Table=|  InternalRulePriority=Speed  RndMeth=Simplest
      BreakpointsForDimension1=|
      | [0; 0.025;
      | 0.051;
      | 0.076;
      | 0.102;
      | 0.127;
      | 0.152;
      | 0.178;
      | 0.203;
      | 0.229;
      | 0.254;
      | 0.279;
      | 0.305
      | ]
      Table=|
      | [0; 35.586;
      | 48.930;
      | 53.379;
      | 53.379;
      | 48.930;
      | 48.930;
      | 48.930;
      | 48.930;
      | 48.930;
      | 48.930;
      | 48.930;
      | 48.930
      | ]
  Saturation : Saturate  UpperLimit=inf  LowerLimit=0
  Saturation1 : Saturate  UpperLimit=0  LowerLimit=-inf
  Subtract : Sum  Inputs=+-
  Subtract1 : Sum  Inputs=+-
  F_RL : Outport
  wires:
  Rear Compression min/1 -> Subtract/2, Add1/2
  Rear Rebound min/1 -> Add2/2, Subtract1/2
  Subtract1/1 -> Gain3/1
  Gain3/1 -> Add2/1
  Subtract/1 -> Gain2/1
  Gain2/1 -> Add1/1
  Rear Compression max/1 -> Subtract/1
  Rear Rebound max/1 -> Subtract1/1
  Saturation/1 -> Rear Compression min/1, Rear Compression max/1
  Gain1/1 -> Rear Rebound min/1, Rear Rebound max/1
  Add2/1 -> Gain/1
  V_RL/1 -> Saturation/1, Saturation1/1
  Saturation1/1 -> Gain1/1
  Gain/1 -> Add/2
  Add1/1 -> Add/1
  Add/1 -> F_RL/1

== system Vehicle_definitivo_validazione_2/Con relaxation/Vehicle/Chassis/Damper/RR ==
  V_RR : Inport
  Add : Sum
  Add1 : Sum
  Add2 : Sum
  Gain : Gain  Gain=-1
  Gain1 : Gain  Gain=-1
  Gain2 : Gain  Gain=car.click_comp_R/car.click_tot_comp_R
  Gain3 : Gain  Gain=car.click_reb_R/car.click_tot_reb_R
  Rear Compression max : Lookup_n-D  NumberOfTableDimensions=1  BreakpointsForDimension1=|  Table=|  InternalRulePriority=Speed  RndMeth=Simplest
      BreakpointsForDimension1=|
      | [0; 0.025;
      | 0.051;
      | 0.076;
      | 0.102;
      | 0.127;
      | 0.152;
      | 0.178;
      | 0.203;
      | 0.229;
      | 0.254;
      | 0.279;
      | 0.305
      | ]
      Table=|
      | [0; 667.233;
      | 782.887;
      | 885.196;
      | 934.126;
      | 965.264;
      | 996.401;
      | 1018.642;
      | 1049.780;
      | 1076.469;
      | 1112.055;
      | 1138.744;  1169.882
      | ]
  Rear Compression min : Lookup_n-D  NumberOfTableDimensions=1  BreakpointsForDimension1=|  Table=|  InternalRulePriority=Speed  RndMeth=Simplest
      BreakpointsForDimension1=|
      | [0; 0.025;
      | 0.051;
      | 0.076;
      | 0.102;
      | 0.127;
      | 0.152;
      | 0.178;
      | 0.203;
      | 0.229;
      | 0.254;
      | 0.279;
      | 0.305
      | ]
      Table=|
      | [0; 213.515;
      | 204.618;
      | 200.170;
      | 195.722;
      | 195.722;
      | 200.170;
      | 200.170;
      | 204.618;
      | 204.618;
      | 209.066;
      | 213.515;
      | 213.515
      | ]
  Rear Rebound max : Lookup_n-D  NumberOfTableDimensions=1  BreakpointsForDimension1=|  Table=|  InternalRulePriority=Speed  RndMeth=Simplest
      BreakpointsForDimension1=|
      | [0; 0.025;
      | 0.051;
      | 0.076;
      | 0.102;
      | 0.127;
      | 0.152;
      | 0.178;
      | 0.203;
      | 0.229;
      | 0.254;
      | 0.279;
      | 0.305
      | ]
      Table=|
      | [0; 124.550;
      | 191.273;
      | 244.652;
      | 284.686;
      | 329.168;
      | 369.202;
      | 391.443;
      | 413.684;
      | 431.477;
      | 449.270;
      | 458.167;
      | 471.511
      | ]
  Rear Rebound min : Lookup_n-D  NumberOfTableDimensions=1  BreakpointsForDimension1=|  Table=|  InternalRulePriority=Speed  RndMeth=Simplest
      BreakpointsForDimension1=|
      | [0; 0.025;
      | 0.051;
      | 0.076;
      | 0.102;
      | 0.127;
      | 0.152;
      | 0.178;
      | 0.203;
      | 0.229;
      | 0.254;
      | 0.279;
      | 0.305
      | ]
      Table=|
      | [0; 35.586;
      | 48.930;
      | 53.379;
      | 53.379;
      | 48.930;
      | 48.930;
      | 48.930;
      | 48.930;
      | 48.930;
      | 48.930;
      | 48.930;
      | 48.930
      | ]
  Saturation : Saturate  UpperLimit=inf  LowerLimit=0
  Saturation1 : Saturate  UpperLimit=0  LowerLimit=-inf
  Subtract : Sum  Inputs=+-
  Subtract1 : Sum  Inputs=+-
  F_RR : Outport
  wires:
  Rear Compression min/1 -> Subtract/2, Add1/2
  Rear Rebound min/1 -> Add2/2, Subtract1/2
  Subtract1/1 -> Gain3/1
  Gain3/1 -> Add2/1
  Subtract/1 -> Gain2/1
  Gain2/1 -> Add1/1
  Rear Compression max/1 -> Subtract/1
  Rear Rebound max/1 -> Subtract1/1
  Saturation/1 -> Rear Compression min/1, Rear Compression max/1
  Gain1/1 -> Rear Rebound min/1, Rear Rebound max/1
  Add2/1 -> Gain/1
  V_RR/1 -> Saturation/1, Saturation1/1
  Saturation1/1 -> Gain1/1
  Gain/1 -> Add/2
  Add1/1 -> Add/1
  Add/1 -> F_RR/1

== system Vehicle_definitivo_validazione_2/Con relaxation/Vehicle/Chassis/kinematics/FL ==
  note: mettere 2d su cmaber e toe
  Steer_Angle : Inport
  Wheel_Travel : Inport  Port=2
  Add : Sum
  Add1 : Sum  Inputs=+++
  Anti_dive : Lookup_n-D  NumberOfTableDimensions=1  BreakpointsForDimension1=[-20;-19;-18;-17;-16;-15;-14;-13;-12;-11;-10;-9;-8;-7;-6;-5;-4;-3;-2;-1;0;1;2;3;4;5;6;7;8;9;10;11;12;13;14;15;16;17;18;19;20;21;22;23;24;25;26;27;28;29;30;31;32;33;34;35;36;37;38;39;40;41;42;43;44;45;46;47;48;49;50;51;52;53;54;55;56;57;58;59;60;61;62;63;64;65;66;67;68;69;70;71;72;73;74;75]  Table=[53.85;54.03;54.22;54.4;54.59;54.77;54.96;55.15;55.34;55.53;55.72;55.92;56.11;56.31;56.5;56.7;56.9;57.1;57.3;57.5;57.71;57.91;58.12;58.32;58.53;58.74;58.95;59.16;59.38;59.59;59.81;60.03;60.24;60.46;60.69;60.91;61.13;61.36;61.59;61.81;62.04;62.28;62.51;62.74;62.98;63.22;63.46;63.7;63.94;64.18000000000001;64.43000000000001;64.68000000000001;64.92;65.17;65.43000000000001;65.68000000000001;65.94;66.19;66.45;66.72;66.98;67.23999999999999;67.51000000000001;67.78;68.05;68.31999999999999;68.59999999999999;68.87;69.15000000000001;69.43000000000001;69.72;70;70.29000000000001;70.58;70.87;71.16;71.45999999999999;71.75;72.05;72.36;72.66;72.97;73.28;73.59;73.91;74.22;74.54000000000001;74.86;75.19;75.52;75.84999999999999;76.18000000000001;76.51000000000001;76.84999999999999;77.19;77.54000000000001]/100  InternalRulePriority=Speed  RndMeth=Simplest
  Constant : Constant  Value=car.camber0_front
  Constant1 : Constant  Value=car.toe0_front
  Gain : Gain  Gain=0.222222
  Gain1 : Gain  Gain=-1
  Gain2 : Gain  Gain=-1
  IR : Lookup_n-D  NumberOfTableDimensions=1  BreakpointsForDimension1=[-20;-19;-18;-17;-16;-15;-14;-13;-12;-11;-10;-9;-8;-7;-6;-5;-4;-3;-2;-1;0;1;2;3;4;5;6;7;8;9;10;11;12;13;14;15;16;17;18;19;20;21;22;23;24;25;26;27;28;29;30;31;32;33;34;35;36;37;38;39;40;41;42;43;44;45;46;47;48;49;50;51;52;53;54;55;56;57;58;59;60;61;62;63;64;65;66;67;68;69;70;71;72;73;74;75]  Table=[0.556793;0.557414;0.558036;0.558659;0.559284;0.55991;0.5602240000000001;0.560538;0.561167;0.561167;0.561482;0.561798;0.562114;0.562114;0.562114;0.562114;0.562114;0.562114;0.562114;0.562114;0.561798;0.561798;0.561482;0.561482;0.561167;0.560852;0.560538;0.5602240000000001;0.55991;0.559284;0.558971;0.558347;0.558036;0.557414;0.557103;0.5564829999999999;0.555864;0.555247;0.554631;0.554017;0.553403;0.552792;0.552181;0.551572;0.550661;0.550055;0.549451;0.548546;0.547945;0.547046;0.546448;0.545554;0.544662;0.543774;0.543183;0.542299;0.541419;0.540541;0.539665;0.538793;0.537924;0.537057;0.536193;0.535332;0.534474;0.533618;0.532765;0.531915;0.531067;0.529942;0.529101;0.528262;0.527426;0.526593;0.525486;0.524659;0.523834;0.522739;0.521921;0.521105;0.5202909999999999;0.519211;0.5184029999999999;0.517598;0.516529;0.51573;0.514933;0.514139;0.513084;0.5122949999999999;0.511509;0.510725;0.509944;0.509165;0.508388;0.507614]  InternalRulePriority=Speed  RndMeth=Simplest
  camber : Lookup_n-D  NumberOfTableDimensions=1  BreakpointsForDimension1=[-20;-19;-18;-17;-16;-15;-14;-13;-12;-11;-10;-9;-8;-7;-6;-5;-4;-3;-2;-1;0;1;2;3;4;5;6;7;8;9;10;11;12;13;14;15;16;17;18;19;20;21;22;23;24;25;26;27;28;29;30;31;32;33;34;35;36;37;38;39;40;41;42;43;44;45;46;47;48;49;50;51;52;53;54;55;56;57;58;59;60;61;62;63;64;65;66;67;68;69;70;71;72;73;74;75]  Table=[0.17;0.13;0.08;0.04;-0.01;-0.05;-0.1;-0.15;-0.19;-0.24;-0.29;-0.33;-0.38;-0.42;-0.47;-0.52;-0.5600000000000001;-0.61;-0.66;-0.7;-0.75;-0.8;-0.84;-0.89;-0.9399999999999999;-0.98;-1.03;-1.08;-1.13;-1.17;-1.22;-1.27;-1.31;-1.36;-1.41;-1.46;-1.5;-1.55;-1.6;-1.65;-1.7;-1.74;-1.79;-1.84;-1.89;-1.94;-1.99;-2.03;-2.08;-2.13;-2.18;-2.23;-2.28;-2.33;-2.38;-2.42;-2.47;-2.52;-2.57;-2.62;-2.67;-2.72;-2.77;-2.82;-2.87;-2.92;-2.97;-3.02;-3.07;-3.12;-3.17;-3.23;-3.28;-3.33;-3.38;-3.43;-3.48;-3.53;-3.58;-3.64;-3.69;-3.74;-3.79;-3.84;-3.9;-3.95;-4;-4.05;-4.11;-4.16;-4.21;-4.27;-4.32;-4.37;-4.43;-4.48]+0.75  InternalRulePriority=Speed  RndMeth=Simplest
  steer vs toe : Lookup_n-D  NumberOfTableDimensions=1  BreakpointsForDimension1=new_lotus_steer.rack_travel  Table=new_lotus_steer.toe_angle_LHS  InternalRulePriority=Speed  RndMeth=Simplest
  toe : Lookup_n-D  NumberOfTableDimensions=1  BreakpointsForDimension1=[-20;-19;-18;-17;-16;-15;-14;-13;-12;-11;-10;-9;-8;-7;-6;-5;-4;-3;-2;-1;0;1;2;3;4;5;6;7;8;9;10;11;12;13;14;15;16;17;18;19;20;21;22;23;24;25;26;27;28;29;30;31;32;33;34;35;36;37;38;39;40;41;42;43;44;45;46;47;48;49;50;51;52;53;54;55;56;57;58;59;60;61;62;63;64;65;66;67;68;69;70;71;72;73;74;75]  Table=new_lotus_bump.front_LHS.toe  InternalRulePriority=Speed  RndMeth=Simplest
  wheelbase_change : Lookup_n-D  NumberOfTableDimensions=1  BreakpointsForDimension1=[-20;-19;-18;-17;-16;-15;-14;-13;-12;-11;-10;-9;-8;-7;-6;-5;-4;-3;-2;-1;0;1;2;3;4;5;6;7;8;9;10;11;12;13;14;15;16;17;18;19;20;21;22;23;24;25;26;27;28;29;30;31;32;33;34;35;36;37;38;39;40;41;42;43;44;45;46;47;48;49;50;51;52;53;54;55;56;57;58;59;60;61;62;63;64;65;66;67;68;69;70;71;72;73;74;75]  Table=[0.68000000000000005;0.65000000000000002;0.60999999999999999;0.56999999999999995;0.54000000000000004;0.5;0.46999999999999997;0.42999999999999999;0.40000000000000002;0.35999999999999999;0.33000000000000002;0.28999999999999998;0.26000000000000001;0.23000000000000001;0.19;0.16;0.13;0.089999999999999997;0.059999999999999998;0.029999999999999999;0;-0.029999999999999999;-0.059999999999999998;-0.089999999999999997;-0.12;-0.14999999999999999;-0.17999999999999999;-0.20999999999999999;-0.23999999999999999;-0.27000000000000002;-0.29999999999999999;-0.32000000000000001;-0.34999999999999998;-0.38;-0.40000000000000002;-0.42999999999999999;-0.46000000000000002;-0.47999999999999998;-0.51000000000000001;-0.53000000000000003;-0.56000000000000005;-0.57999999999999996;-0.60999999999999999;-0.63;-0.65000000000000002;-0.68000000000000005;-0.69999999999999996;-0.71999999999999997;-0.73999999999999999;-0.76000000000000001;-0.79000000000000004;-0.81000000000000005;-0.82999999999999996;-0.84999999999999998;-0.87;-0.89000000000000001;-0.91000000000000003;-0.92000000000000004;-0.93999999999999995;-0.95999999999999996;-0.97999999999999998;-0.98999999999999999;-1.01;-1.03;-1.04;-1.0600000000000001;-1.0700000000000001;-1.0900000000000001;-1.1000000000000001;-1.1200000000000001;-1.1299999999999999;-1.1399999999999999;-1.1499999999999999;-1.1699999999999999;-1.1799999999999999;-1.1899999999999999;-1.2;-1.21;-1.22;-1.23;-1.24;-1.25;-1.26;-1.26;-1.27;-1.28;-1.29;-1.29;-1.3;-1.3;-1.3100000000000001;-1.3100000000000001;-1.3100000000000001;-1.3200000000000001;-1.3200000000000001;-1.3200000000000001]/1000  InternalRulePriority=Speed  RndMeth=Simplest
  wb_FL : Outport
  AD_FL : Outport  Port=2
  IR_FL : Outport  Port=3
  Camber_FL : Outport  Port=4
  Toe_FL : Outport  Port=5
  wires:
  Wheel_Travel/1 -> Anti_dive/1, IR/1, camber/1, toe/1, wheelbase_change/1
  wheelbase_change/1 -> wb_FL/1
  Anti_dive/1 -> AD_FL/1
  IR/1 -> IR_FL/1
  Constant1/1 -> Add1/1
  Add/1 -> Camber_FL/1
  camber/1 -> Add/2
  Add1/1 -> Toe_FL/1
  Constant/1 -> Add/1
  toe/1 -> Gain2/1
  Steer_Angle/1 -> Gain/1
  Gain/1 -> steer vs toe/1
  steer vs toe/1 -> Gain1/1  "toe_FL"
  Gain1/1 -> Add1/3
  Gain2/1 -> Add1/2
